simulink model "kundur_two_area_system_open_control"  (R2019a)
settings: Solver=VariableStepAuto  StartTime=0.0  StopTime=40  RelTol=1e-3
libraries: powerlib x43, powerlib_meascontrol x3
settings Model: Creator=Ram Baskar  LastModifiedBy=Ram Baskar

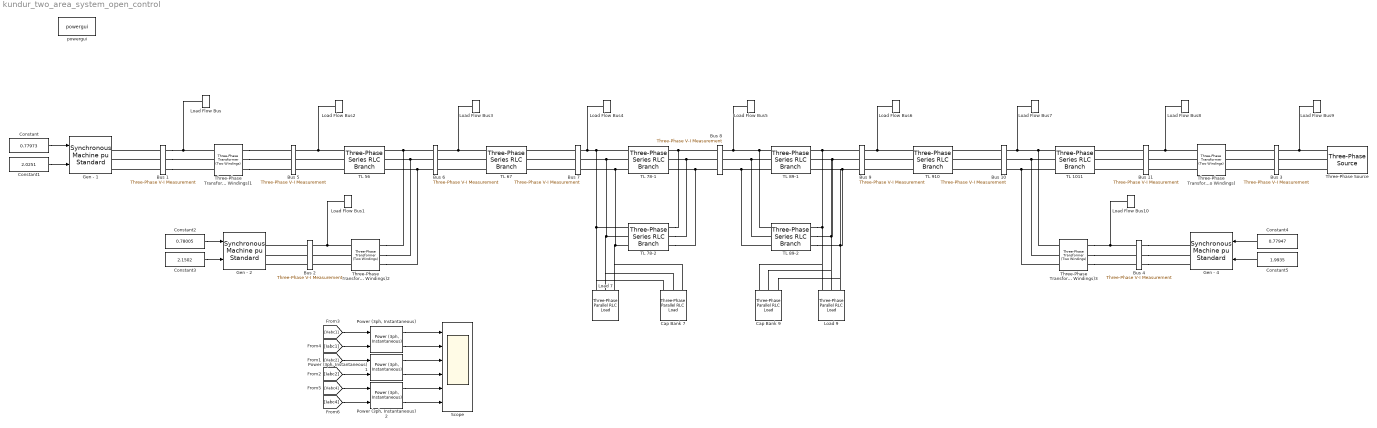
== system kundur_two_area_system_open_control ==
  Bus 1 : powerlib/Measurements/Three-Phase V-I Measurement  VoltageMeasurement=phase-to-ground  SetLabelV=on  LabelV=Vabc1  Vpu=off  VpuLL=off  CurrentMeasurement=yes  SetLabelI=on  LabelI=Iabc1  Ipu=off  Pbase=100e6  Vbase=500e3  OutputType=Complex  PhasorSimulation=off  PSBequivalent=0
      settings: SourceProductName=Simscape Electrical
  Bus 10 : powerlib/Measurements/Three-Phase V-I Measurement  VoltageMeasurement=phase-to-ground  SetLabelV=on  LabelV=Vabc10  Vpu=off  VpuLL=off  CurrentMeasurement=yes  SetLabelI=on  LabelI=Iabc10  Ipu=off  Pbase=100e6  Vbase=500e3  OutputType=Complex  PhasorSimulation=off  PSBequivalent=0
      settings: SourceProductName=Simscape Electrical
  Bus 11 : powerlib/Measurements/Three-Phase V-I Measurement  VoltageMeasurement=phase-to-ground  SetLabelV=on  LabelV=Vabc11  Vpu=off  VpuLL=off  CurrentMeasurement=yes  SetLabelI=on  LabelI=Iabc11  Ipu=off  Pbase=100e6  Vbase=500e3  OutputType=Complex  PhasorSimulation=off  PSBequivalent=0
      settings: SourceProductName=Simscape Electrical
  Bus 2 : powerlib/Measurements/Three-Phase V-I Measurement  VoltageMeasurement=phase-to-ground  SetLabelV=on  LabelV=Vabc2  Vpu=off  VpuLL=off  CurrentMeasurement=yes  SetLabelI=on  LabelI=Iabc2  Ipu=off  Pbase=100e6  Vbase=500e3  OutputType=Complex  PhasorSimulation=off  PSBequivalent=0
      settings: SourceProductName=Simscape Electrical
  Bus 3 : powerlib/Measurements/Three-Phase V-I Measurement  VoltageMeasurement=phase-to-ground  SetLabelV=on  LabelV=Vabc3  Vpu=off  VpuLL=off  CurrentMeasurement=yes  SetLabelI=on  LabelI=Iabc3  Ipu=off  Pbase=100e6  Vbase=500e3  OutputType=Complex  PhasorSimulation=off  PSBequivalent=0
      settings: SourceProductName=Simscape Electrical
  Bus 4 : powerlib/Measurements/Three-Phase V-I Measurement  VoltageMeasurement=phase-to-ground  SetLabelV=on  LabelV=Vabc4  Vpu=off  VpuLL=off  CurrentMeasurement=yes  SetLabelI=on  LabelI=Iabc4  Ipu=off  Pbase=100e6  Vbase=500e3  OutputType=Complex  PhasorSimulation=off  PSBequivalent=0
      settings: SourceProductName=Simscape Electrical
  Bus 5 : powerlib/Measurements/Three-Phase V-I Measurement  VoltageMeasurement=phase-to-ground  SetLabelV=on  LabelV=Vabc5  Vpu=off  VpuLL=off  CurrentMeasurement=yes  SetLabelI=on  LabelI=Iabc5  Ipu=off  Pbase=100e6  Vbase=500e3  OutputType=Complex  PhasorSimulation=off  PSBequivalent=0
      settings: SourceProductName=Simscape Electrical
  Bus 6 : powerlib/Measurements/Three-Phase V-I Measurement  VoltageMeasurement=phase-to-ground  SetLabelV=on  LabelV=Vabc6  Vpu=off  VpuLL=off  CurrentMeasurement=yes  SetLabelI=on  LabelI=Iabc6  Ipu=off  Pbase=100e6  Vbase=500e3  OutputType=Complex  PhasorSimulation=off  PSBequivalent=0
      settings: SourceProductName=Simscape Electrical
  Bus 7 : powerlib/Measurements/Three-Phase V-I Measurement  VoltageMeasurement=phase-to-ground  SetLabelV=on  LabelV=Vabc7  Vpu=off  VpuLL=off  CurrentMeasurement=yes  SetLabelI=on  LabelI=Iabc7  Ipu=off  Pbase=100e6  Vbase=500e3  OutputType=Complex  PhasorSimulation=off  PSBequivalent=0
      settings: SourceProductName=Simscape Electrical
  Bus 8 : powerlib/Measurements/Three-Phase V-I Measurement  VoltageMeasurement=phase-to-ground  SetLabelV=on  LabelV=Vabc8  Vpu=off  VpuLL=off  CurrentMeasurement=yes  SetLabelI=on  LabelI=Iabc8  Ipu=off  Pbase=100e6  Vbase=500e3  OutputType=Complex  PhasorSimulation=off  PSBequivalent=0
      settings: SourceProductName=Simscape Electrical
  Bus 9 : powerlib/Measurements/Three-Phase V-I Measurement  VoltageMeasurement=phase-to-ground  SetLabelV=on  LabelV=Vabc9  Vpu=off  VpuLL=off  CurrentMeasurement=yes  SetLabelI=on  LabelI=Iabc9  Ipu=off  Pbase=100e6  Vbase=500e3  OutputType=Complex  PhasorSimulation=off  PSBequivalent=0
      settings: SourceProductName=Simscape Electrical
  Cap Bank 7 : powerlib/Elements/Three-Phase Parallel RLC Load  LConnTagsString=A|B|C  Configuration=Y (grounded)  NominalVoltage=230e3*0.8958  Vabc=[1e3 1e3 1e3]  Vabcp=[1e3 1e3 1e3]  NominalFrequency=60  UnbalancedPower=off  ActivePower=0  InductivePower=0  CapacitivePower=200e6  Pabc=[10e3 9e3 11e3]  QLabc=[100 90 110]  QCabc=[100 90 110]  Pabcp=[10e3 9e3 11e3]  QLabcp=[100 90 110]  QCabcp=[100 90 110]  Measurements=Branch voltages and currents  LoadType=constant Z
      settings: SourceProductName=Simscape Electrical
  Cap Bank 9 : powerlib/Elements/Three-Phase Parallel RLC Load  LConnTagsString=A|B|C  Configuration=Y (grounded)  NominalVoltage=230e3*0.9667  Vabc=[1e3 1e3 1e3]  Vabcp=[1e3 1e3 1e3]  NominalFrequency=60  UnbalancedPower=off  ActivePower=0  InductivePower=0  CapacitivePower=350e6  Pabc=[10e3 9e3 11e3]  QLabc=[100 90 110]  QCabc=[100 90 110]  Pabcp=[10e3 9e3 11e3]  QLabcp=[100 90 110]  QCabcp=[100 90 110]  Measurements=Branch voltages and currents  LoadType=constant Z
      settings: SourceProductName=Simscape Electrical
  Constant : Constant  Value=0.77973
  Constant1 : Constant  Value=2.0251
  Constant2 : Constant  Value=0.78005
  Constant3 : Constant  Value=2.1502
  Constant4 : Constant  Value=0.77947
  Constant5 : Constant  Value=1.9935
  Gen - 1 : powerlib/Machines/Synchronous Machine pu Standard  PresetModel=No  MechanicalLoad=Mechanical power Pm  ShowDetailedParameters=on  RotorType=Round  Units=per unit standard parameters  MeasurementBus=off  NominalParameters=[900e6 20e3 60]  Reactances1=[ 1.80 0.30 0.25 1.70 0.55 0.25 0.20 ]  Reactances2=[2.24 0.17 0.12 1.02 0.13 0.08]  dAxisTimeConstants=Open-circuit  qAxisTimeConstants=Open-circuit  TimeConstants1="[ 4.4849  0.0681  0.1  ]"  TimeConstants2=[ 8.0 0.03 0.40 0.05 ]  TimeConstants3="[  4.49  0.0681  0.0513  ]"  TimeConstants4=[ 8.0, 0.03, 0.3371, 0.0295 ]  TimeConstants5=[ 1.01, 0.053, 0.1 ]  TimeConstants6=[ 1.3201, 0.023, 1.0, 0.07 ]  TimeConstants7=[0.012 0.003 0.003]  TimeConstants8=[ 1.3201, 0.0231, 0.3371, 0.0295 ]  StatorResistance=0.0025  Mechanical=[6.50 0.02 1]  PolePairs=20  InitialConditions=[0 12.9481 0.883667 0.883667 0.883667 39.9069 -80.0931 159.907 2.02512]  SetSaturation=off  Saturation=[0.6404,0.7127,0.8441,0.9214,0.9956,1.082,1.19,1.316,1.457;0.7,0.7698,0.8872,0.9466,0.9969,1.046,1.1,1.151,1.201]  LoadFlowParameters=[1,0,0,0,0]  TsPowergui=0  TsBlock=-1  IterativeModel=Trapezoidal non iterative  IterativeDiscreteModel=Trapezoidal non iterative  BusType=PQ  Pref=700e6  Qref=185e6  Qmin=-inf  Qmax=inf  PLF=0  QLF=0
      settings: SourceProductName=Simscape Electrical
  Gen - 2 : powerlib/Machines/Synchronous Machine pu Standard  PresetModel=No  MechanicalLoad=Mechanical power Pm  ShowDetailedParameters=on  RotorType=Round  Units=per unit standard parameters  MeasurementBus=off  NominalParameters=[900e6 20e3 60]  Reactances1=[ 1.80 0.30 0.25 1.70 0.55 0.25 0.20 ]  Reactances2=[2.24 0.17 0.12 1.02 0.13 0.08]  dAxisTimeConstants=Open-circuit  qAxisTimeConstants=Open-circuit  TimeConstants1="[ 4.4849  0.0681  0.1  ]"  TimeConstants2=[ 8.0, 0.03, 0.40, 0.05 ]  TimeConstants3="[  4.49  0.0681  0.0513  ]"  TimeConstants4=[ 8.0, 0.03, 0.3371, 0.0295 ]  TimeConstants5=[ 1.01, 0.053, 0.1 ]  TimeConstants6=[ 1.3201, 0.023, 1.0, 0.07 ]  TimeConstants7=[0.012 0.003 0.003]  TimeConstants8=[ 1.3201, 0.0231, 0.3371, 0.0295 ]  StatorResistance=0.0025  Mechanical=[6.50 0.02 1]  PolePairs=20  InitialConditions=[0 0.23842 0.952429 0.952429 0.952429 23.631 -96.369 143.631 2.15025]  SetSaturation=off  Saturation=[0.6404,0.7127,0.8441,0.9214,0.9956,1.082,1.19,1.316,1.457;0.7,0.7698,0.8872,0.9466,0.9969,1.046,1.1,1.151,1.201]  LoadFlowParameters=[1,0,0,0,0]  TsPowergui=0  TsBlock=-1  IterativeModel=Trapezoidal non iterative  IterativeDiscreteModel=Trapezoidal non iterative  BusType=PQ  Pref=700e6  Qref=235e6  Qmin=-inf  Qmax=inf  PLF=0  QLF=0
      settings: SourceProductName=Simscape Electrical
  Gen - 4 : powerlib/Machines/Synchronous Machine pu Standard  PresetModel=No  MechanicalLoad=Mechanical power Pm  ShowDetailedParameters=on  RotorType=Round  Units=per unit standard parameters  MeasurementBus=off  NominalParameters=[900e6 20e3 60]  Reactances1=[ 1.80 0.30 0.25 1.70 0.55 0.25 0.20 ]  Reactances2=[2.24 0.17 0.12 1.02 0.13 0.08]  dAxisTimeConstants=Open-circuit  qAxisTimeConstants=Open-circuit  TimeConstants1="[ 4.4849  0.0681  0.1  ]"  TimeConstants2=[ 8.0, 0.03, 0.40, 0.05 ]  TimeConstants3="[  4.49  0.0681  0.0513  ]"  TimeConstants4=[ 8.0, 0.03, 0.3371, 0.0295 ]  TimeConstants5=[ 1.01, 0.053, 0.1 ]  TimeConstants6=[ 1.3201, 0.023, 1.0, 0.07 ]  TimeConstants7=[0.012 0.003 0.003]  TimeConstants8=[ 1.3201, 0.0231, 0.3371, 0.0295 ]  StatorResistance=0.0025  Mechanical=[6.175 0.02 1]  PolePairs=20  InitialConditions=[0 -53.1021 0.823597 0.823597 0.823597 -23.5996 -143.6 96.4004 1.99351]  SetSaturation=off  Saturation=[0.6404,0.7127,0.8441,0.9214,0.9956,1.082,1.19,1.316,1.457;0.7,0.7698,0.8872,0.9466,0.9969,1.046,1.1,1.151,1.201]  LoadFlowParameters=[1,0,0,0,0]  TsPowergui=0  TsBlock=-1  IterativeModel=Trapezoidal non iterative  IterativeDiscreteModel=Trapezoidal non iterative  BusType=PQ  Pref=700e6  Qref=202e6  Qmin=-inf  Qmax=inf  PLF=0  QLF=0
      settings: SourceProductName=Simscape Electrical
  "Load 7 " : powerlib/Elements/Three-Phase Parallel RLC Load  LConnTagsString=A|B|C  Configuration=Y (grounded)  NominalVoltage=230e3*0.8958  Vabc=[1e3 1e3 1e3]  Vabcp=[1e3 1e3 1e3]  NominalFrequency=60  UnbalancedPower=off  ActivePower=967e6  InductivePower=100e6  CapacitivePower=0  Pabc=[10e3 9e3 11e3]  QLabc=[100 90 110]  QCabc=[100 90 110]  Pabcp=[10e3 9e3 11e3]  QLabcp=[100 90 110]  QCabcp=[100 90 110]  Measurements=Branch voltages and currents  LoadType=constant Z
      settings: SourceProductName=Simscape Electrical
  "Load 9 " : powerlib/Elements/Three-Phase Parallel RLC Load  LConnTagsString=A|B|C  Configuration=Y (grounded)  NominalVoltage=230e3*0.9667  Vabc=[1e3 1e3 1e3]  Vabcp=[1e3 1e3 1e3]  NominalFrequency=60  UnbalancedPower=off  ActivePower=1767e6  InductivePower=100e6  CapacitivePower=0  Pabc=[10e3 9e3 11e3]  QLabc=[100 90 110]  QCabc=[100 90 110]  Pabcp=[10e3 9e3 11e3]  QLabcp=[100 90 110]  QCabcp=[100 90 110]  Measurements=Branch voltages and currents  LoadType=constant Z
      settings: SourceProductName=Simscape Electrical
  Load Flow Bus : powerlib/Measurements/Load Flow Bus  LConnTagsString=a  Phases=single  Connectors=on one side  ID=BUS_1  Vbase=20e3  Vref=1  Vangle=0  VLF=0.9104  VLFb=1  VLFc=1  angleLF=54.71  angleLFb=0  angleLFc=0
      settings: SourceProductName=Simscape Electrical
  Load Flow Bus1 : powerlib/Measurements/Load Flow Bus  LConnTagsString=a  Phases=single  Connectors=on one side  ID=BUS_2  Vbase=20e3  Vref=1  Vangle=0  VLF=0.8614  VLFb=1  VLFc=1  angleLF=42.19  angleLFb=0  angleLFc=0
      settings: SourceProductName=Simscape Electrical
  Load Flow Bus10 : powerlib/Measurements/Load Flow Bus  LConnTagsString=a  Phases=single  Connectors=on one side  ID=BUS_4  Vbase=20e3  Vref=1  Vangle=0  VLF=0.9829  VLFb=1  VLFc=1  angleLF=-7.503  angleLFb=0  angleLFc=0
      settings: SourceProductName=Simscape Electrical
  Load Flow Bus2 : powerlib/Measurements/Load Flow Bus  LConnTagsString=a  Phases=single  Connectors=on one side  ID=BUS_5  Vbase=230e3  Vref=1  Vangle=0  VLF=0.9103  VLFb=1  VLFc=1  angleLF=54.69  angleLFb=0  angleLFc=0
      settings: SourceProductName=Simscape Electrical
  Load Flow Bus3 : powerlib/Measurements/Load Flow Bus  LConnTagsString=a  Phases=single  Connectors=on one side  ID=BUS_6  Vbase=230e3  Vref=1  Vangle=0  VLF=0.8613  VLFb=1  VLFc=1  angleLF=42.16  angleLFb=0  angleLFc=0
      settings: SourceProductName=Simscape Electrical
  Load Flow Bus4 : powerlib/Measurements/Load Flow Bus  LConnTagsString=a  Phases=single  Connectors=on one side  ID=BUS_7  Vbase=230e3  Vref=1  Vangle=0  VLF=0.8302  VLFb=1  VLFc=1  angleLF=31.24  angleLFb=0  angleLFc=0
      settings: SourceProductName=Simscape Electrical
  Load Flow Bus5 : powerlib/Measurements/Load Flow Bus  LConnTagsString=a  Phases=single  Connectors=on one side  ID=BUS_8  Vbase=230e3  Vref=1  Vangle=0  VLF=0.8181  VLFb=1  VLFc=1  angleLF=6.519  angleLFb=0  angleLFc=0
      settings: SourceProductName=Simscape Electrical
  Load Flow Bus6 : powerlib/Measurements/Load Flow Bus  LConnTagsString=a  Phases=single  Connectors=on one side  ID=BUS_9  Vbase=230e3  Vref=1  Vangle=0  VLF=0.948  VLFb=1  VLFc=1  angleLF=-14.96  angleLFb=0  angleLFc=0
      settings: SourceProductName=Simscape Electrical
  Load Flow Bus7 : powerlib/Measurements/Load Flow Bus  LConnTagsString=a  Phases=single  Connectors=on one side  ID=BUS_10  Vbase=230e3  Vref=1  Vangle=0  VLF=0.9828  VLFb=1  VLFc=1  angleLF=-7.521  angleLFb=0  angleLFc=0
      settings: SourceProductName=Simscape Electrical
  Load Flow Bus8 : powerlib/Measurements/Load Flow Bus  LConnTagsString=a  Phases=single  Connectors=on one side  ID=BUS_11  Vbase=230e3  Vref=1  Vangle=0  VLF=1.03  VLFb=1  VLFc=1  angleLF=-0.01307  angleLFb=0  angleLFc=0
      settings: SourceProductName=Simscape Electrical
  Load Flow Bus9 : powerlib/Measurements/Load Flow Bus  LConnTagsString=a  Phases=single  Connectors=on one side  ID=BUS_3  Vbase=20e3  Vref=1.03  Vangle=0  VLF=1.03  VLFb=1  VLFc=1  angleLF=0  angleLFb=0  angleLFc=0
      settings: SourceProductName=Simscape Electrical
  "Power (3ph, Instantaneous)" : powerlib_meascontrol/Measurements/Power (3ph, Instantaneous)
      settings: SourceProductName=Simscape Electrical
  "Power (3ph, Instantaneous)1" : powerlib_meascontrol/Measurements/Power (3ph, Instantaneous)
      settings: SourceProductName=Simscape Electrical
  "Power (3ph, Instantaneous)2" : powerlib_meascontrol/Measurements/Power (3ph, Instantaneous)
      settings: SourceProductName=Simscape Electrical
  Scope : Scope  NumInputPorts=6
  TL 1011 : powerlib/Elements/Three-Phase Series RLC Branch  LConnTagsString=A|B|C  RConnTagsString=A|B|C  BranchType=RL  Resistance=1.3225  Inductance=0.035080402  Capacitance=1e-6  Measurements=None
      settings: SourceProductName=Simscape Electrical
  TL 56 : powerlib/Elements/Three-Phase Series RLC Branch  LConnTagsString=A|B|C  RConnTagsString=A|B|C  BranchType=RL  Resistance=1.3225  Inductance=0.035080402  Capacitance=1e-6  Measurements=None
      settings: SourceProductName=Simscape Electrical
  "TL 67 " : powerlib/Elements/Three-Phase Series RLC Branch  LConnTagsString=A|B|C  RConnTagsString=A|B|C  BranchType=RL  Resistance=0.529  Inductance=1.403e-02  Capacitance=1e-6  Measurements=None
      settings: SourceProductName=Simscape Electrical
  TL 78-1 : powerlib/Elements/Three-Phase Series RLC Branch  LConnTagsString=A|B|C  RConnTagsString=A|B|C  BranchType=RL  Resistance=5.819  Inductance=1.5443e-01  Capacitance=1e-6  Measurements=None
      settings: SourceProductName=Simscape Electrical
  TL 78-2 : powerlib/Elements/Three-Phase Series RLC Branch  LConnTagsString=A|B|C  RConnTagsString=A|B|C  BranchType=RL  Resistance=5.819  Inductance=1.5443e-01  Capacitance=1e-6  Measurements=None
      settings: SourceProductName=Simscape Electrical
  TL 89-1 : powerlib/Elements/Three-Phase Series RLC Branch  LConnTagsString=A|B|C  RConnTagsString=A|B|C  BranchType=RL  Resistance=5.819  Inductance=1.5443e-01  Capacitance=1e-6  Measurements=None
      settings: SourceProductName=Simscape Electrical
  TL 89-2 : powerlib/Elements/Three-Phase Series RLC Branch  LConnTagsString=A|B|C  RConnTagsString=A|B|C  BranchType=RL  Resistance=5.819  Inductance=1.5443e-01  Capacitance=1e-6  Measurements=None
      settings: SourceProductName=Simscape Electrical
  "TL 910 " : powerlib/Elements/Three-Phase Series RLC Branch  LConnTagsString=A|B|C  RConnTagsString=A|B|C  BranchType=RL  Resistance=0.529  Inductance=1.403e-02  Capacitance=1e-6  Measurements=None
      settings: SourceProductName=Simscape Electrical
  Three-Phase Transformer (Two Windings){,1..3} (4 alike) : powerlib/Elements/Three-Phase Transformer (Two Windings)  Winding1Connection=Yg  Winding2Connection=Yg  CoreType=Three single-phase transformers  SetSaturation=off  Hysteresis=off  DataFile='hysteresis'  SetInitialFlux=off  Measurements=None  UNITS=pu  NominalPower=[ 900e6 , 60 ]  Winding1=[20e3 , 0 , 0.000198944 ]  Winding2=[ 230e3 , 0 , 0.000198944 ]  Rm=500  Lm=500  L0=0.5  Saturation=[ 0,0 ; 0.0024,1.2 ; 1.0,1.52 ]  InitialFluxes=[ 0.8 , -0.8 , 0.7 ]  BreakLoop=off  DiscreteSolver=Trapezoidal iterative  DataType=off  TransfoNumber=1
      settings: SourceProductName=Simscape Electrical
  Three-Phase Source : powerlib/Electrical Sources/Three-Phase Source  InternalConnection=Yg  VoltagePhases=off  Voltage=(20000)*1.03  PhaseAngle=0  Voltage_phases=[25e3 25e3 25e3]/sqrt(3)  PhaseAngles_phases=[0 -120 +120]  Frequency=60  NonIdealSource=off  SpecifyImpedance=off  Resistance=0.8929  Inductance=16.58e-3  ShortCircuitLevel=100e6  BaseVoltage=25e3  XRratio=7  BusType=swing  Pref=10e3  Qref=0  Prefabc=[10e3, 10e3, 10e3]  Qrefabc=[0, 0, 0]  Qmin=-inf  Qmax=inf
      settings: SourceProductName=Simscape Electrical
  powergui : powerlib/powergui  Priority=1  SimulationMode=Discrete  SampleTime=50e-6  frequency=60  Iterations=1000  frequencyindice=60  Pbase=100e6  ErrMax=0.0001  UnitsV=kV  UnitsW=MW  buscounter=0  FunctionMessages=off  echomessages=off  EnableUseOfTLC=off  CurrentSourceSwitches=off  DisableSnubberDevices=off  DisableRonSwitches=off  DisableVfSwitches=off  DisplayEquations=off  AutomaticDiscreteSolvers=on  SolverType=Tustin/Backward Euler (TBE)  Interpol=off  ExternalGateDelay=off  methode=off  Ts=100  x0status=blocks  SPID=on  SwTol=0  HookPort=off  NonlinearTolerance=0  nMaxIteration=15  ContinueOnMaxIteration=off  RestoreLinks=warning  ResistiveCurrentMeasurement=off  Frange=[0:2:500]  Ylog=off  Xlog=on  ShowGrid=off  save=off  variable=ZData  structure=0  ZoomFFT=off  StartTime=0.0  cycles=1  DisplayStyle=1  fundamental=60  FreqAxis=off  MaxFrequency=1000  frequencyindicesteady=1  RmsSteady=1  display=off
      settings: SourceProductName=Simscape Electrical
  wires:
  [Vabc1] -> "Power (3ph, Instantaneous)"/1
  [Iabc1] -> "Power (3ph, Instantaneous)"/2
  "Power (3ph, Instantaneous)"/1 -> Scope/1
  "Power (3ph, Instantaneous)"/2 -> Scope/2
  Constant/1 -> Gen - 1/1
  Constant1/1 -> Gen - 1/2
  Constant2/1 -> Gen - 2/1
  Constant3/1 -> Gen - 2/2
  Constant5/1 -> Gen - 4/2
  Constant4/1 -> Gen - 4/1
  [Iabc2] -> "Power (3ph, Instantaneous)1"/2
  [Vabc2] -> "Power (3ph, Instantaneous)1"/1
  [Iabc4] -> "Power (3ph, Instantaneous)2"/2
  [Vabc4] -> "Power (3ph, Instantaneous)2"/1
  "Power (3ph, Instantaneous)1"/1 -> Scope/3
  "Power (3ph, Instantaneous)1"/2 -> Scope/4
  "Power (3ph, Instantaneous)2"/1 -> Scope/5
  "Power (3ph, Instantaneous)2"/2 -> Scope/6
  connections:
  Bus 1/RConn1 -- Load Flow Bus/LConn1 -- Three-Phase Transformer (Two Windings)1/LConn1
  Bus 1/RConn2 -- Three-Phase Transformer (Two Windings)1/LConn2
  Bus 1/RConn3 -- Three-Phase Transformer (Two Windings)1/LConn3
  Bus 1/LConn2 -- Gen - 1/RConn2
  Bus 1/LConn3 -- Gen - 1/RConn3
  Bus 1/LConn1 -- Gen - 1/RConn1
  TL 56/LConn1 -- Load Flow Bus2/LConn1 -- Bus 5/RConn1
  TL 56/LConn2 -- Bus 5/RConn2
  TL 56/LConn3 -- Bus 5/RConn3
  Three-Phase Transformer (Two Windings)1/RConn2 -- Bus 5/LConn2
  Three-Phase Transformer (Two Windings)1/RConn3 -- Bus 5/LConn3
  Three-Phase Transformer (Two Windings)1/RConn1 -- Bus 5/LConn1
  Bus 6/LConn1 -- Three-Phase Transformer (Two Windings)2/RConn1 -- TL 56/RConn1
  Bus 6/LConn2 -- Three-Phase Transformer (Two Windings)2/RConn2 -- TL 56/RConn2
  Bus 6/LConn3 -- Three-Phase Transformer (Two Windings)2/RConn3 -- TL 56/RConn3
  "TL 67 "/LConn2 -- Bus 6/RConn2
  "TL 67 "/LConn3 -- Bus 6/RConn3
  "TL 67 "/LConn1 -- Load Flow Bus3/LConn1 -- Bus 6/RConn1
  Bus 7/LConn3 -- "TL 67 "/RConn3
  Bus 7/LConn1 -- "TL 67 "/RConn1
  Bus 7/LConn2 -- "TL 67 "/RConn2
  TL 78-1/LConn1 -- Cap Bank 7/LConn1 -- "Load 7 "/LConn1 -- TL 78-2/LConn1 -- Load Flow Bus4/LConn1 -- Bus 7/RConn1
  TL 78-1/LConn2 -- Cap Bank 7/LConn2 -- "Load 7 "/LConn2 -- TL 78-2/LConn2 -- Bus 7/RConn2
  TL 78-1/LConn3 -- Cap Bank 7/LConn3 -- "Load 7 "/LConn3 -- TL 78-2/LConn3 -- Bus 7/RConn3
  Bus 8/LConn1 -- TL 78-2/RConn1 -- TL 78-1/RConn1
  Bus 8/LConn2 -- TL 78-2/RConn2 -- TL 78-1/RConn2
  Bus 8/LConn3 -- TL 78-2/RConn3 -- TL 78-1/RConn3
  TL 89-1/LConn1 -- TL 89-2/LConn1 -- Load Flow Bus5/LConn1 -- Bus 8/RConn1
  TL 89-1/LConn2 -- TL 89-2/LConn2 -- Bus 8/RConn2
  TL 89-1/LConn3 -- TL 89-2/LConn3 -- Bus 8/RConn3
  Bus 9/LConn1 -- TL 89-1/RConn1 -- Cap Bank 9/LConn1 -- "Load 9 "/LConn1 -- TL 89-2/RConn1
  Bus 9/LConn2 -- Cap Bank 9/LConn2 -- "Load 9 "/LConn2 -- TL 89-2/RConn2 -- TL 89-1/RConn2
  Bus 9/LConn3 -- Cap Bank 9/LConn3 -- "Load 9 "/LConn3 -- TL 89-2/RConn3 -- TL 89-1/RConn3
  "TL 910 "/LConn1 -- Load Flow Bus6/LConn1 -- Bus 9/RConn1
  "TL 910 "/LConn2 -- Bus 9/RConn2
  "TL 910 "/LConn3 -- Bus 9/RConn3
  Bus 10/LConn1 -- "TL 910 "/RConn1
  Bus 10/LConn2 -- "TL 910 "/RConn2
  Bus 10/LConn3 -- "TL 910 "/RConn3
  TL 1011/LConn1 -- Three-Phase Transformer (Two Windings)3/RConn1 -- Load Flow Bus7/LConn1 -- Bus 10/RConn1
  TL 1011/LConn2 -- Three-Phase Transformer (Two Windings)3/RConn2 -- Bus 10/RConn2
  TL 1011/LConn3 -- Three-Phase Transformer (Two Windings)3/RConn3 -- Bus 10/RConn3
  Bus 11/LConn1 -- TL 1011/RConn1
  Bus 11/LConn2 -- TL 1011/RConn2
  Bus 11/LConn3 -- TL 1011/RConn3
  Three-Phase Transformer (Two Windings)/RConn1 -- Load Flow Bus8/LConn1 -- Bus 11/RConn1
  Three-Phase Transformer (Two Windings)/RConn2 -- Bus 11/RConn2
  Three-Phase Transformer (Two Windings)/RConn3 -- Bus 11/RConn3
  Bus 3/LConn1 -- Three-Phase Transformer (Two Windings)/LConn1
  Bus 3/LConn2 -- Three-Phase Transformer (Two Windings)/LConn2
  Bus 3/LConn3 -- Three-Phase Transformer (Two Windings)/LConn3
  Three-Phase Source/RConn1 -- Load Flow Bus9/LConn1 -- Bus 3/RConn1
  Three-Phase Source/RConn2 -- Bus 3/RConn2
  Three-Phase Source/RConn3 -- Bus 3/RConn3
  Bus 2/LConn2 -- Gen - 2/RConn2
  Bus 2/LConn1 -- Gen - 2/RConn1
  Bus 2/LConn3 -- Gen - 2/RConn3
  Three-Phase Transformer (Two Windings)2/LConn1 -- Load Flow Bus1/LConn1 -- Bus 2/RConn1
  Three-Phase Transformer (Two Windings)2/LConn2 -- Bus 2/RConn2
  Three-Phase Transformer (Two Windings)2/LConn3 -- Bus 2/RConn3
  Bus 4/LConn1 -- Gen - 4/RConn1
  Bus 4/LConn3 -- Gen - 4/RConn3
  Bus 4/LConn2 -- Gen - 4/RConn2
  Three-Phase Transformer (Two Windings)3/LConn1 -- Load Flow Bus10/LConn1 -- Bus 4/RConn1
  Three-Phase Transformer (Two Windings)3/LConn3 -- Bus 4/RConn3
  Three-Phase Transformer (Two Windings)3/LConn2 -- Bus 4/RConn2
